simulink model "MissionManager"  (R2025b)
settings: Solver=FixedStepDiscrete  StartTime=0.0  StopTime=10  FixedStep=CMD_SAMPLE_TIME  RelTol=1e-3
undefined symbols (not defined in the file): CMD_SAMPLE_TIME
settings Model: DataDictionary=CommandDict.sldd  Creator=89447  LastModifiedBy=89447
settings OptimizationCC: DefaultParameterBehavior=Inlined  EnhancedBackFolding=on  PassReuseOutputArgsAs=Individual arguments  ZeroExternalMemoryAtStartup=off  ZeroInternalMemoryAtStartup=off  MaxStackSize=64  OptimizeBlockOrder=speed  DifferentSizesBufferReuse=on  OptimizationCustomize=off  EfficientTunableParamExpr=on
settings HardwareCC: ProdBitPerLong=64.0  ProdHWDeviceType=Intel->x86-64 (Linux 64)  TargetBitPerLong=64.0  TargetBitPerPointer=64.0  TargetBitPerSizeT=64.0  TargetBitPerPtrDiffT=64.0  TargetLargestAtomicFloat=Float  TargetIntDivRoundTo=Zero  TargetEndianess=LittleEndian  TargetWordSize=64.0  TargetHWDeviceType=Intel->x86-64 (Linux 64)  ProdEqTarget=off
settings SFSimCC: MATLABDynamicMemAlloc=off
settings RTWCC: SystemTargetFile=ert.tlc  HardwareBoard=Robot Operating System 2 (ROS 2)  TLCOptions="-aInlineSetEventsForThisBaseRateFcn=TLC_FALSE -aSuppressMultiTaskScheduler=TLC_FALSE  -aRateBasedStepFcn=0"  TemplateMakefile=ert_default_tmf  Toolchain=Colcon Tools  TargetLang=C++  Description=Embedded Coder
settings CodeAppCC: ForceParamTrailComments=on  IgnoreCustomStorageClasses=off  OperatorAnnotations=on  SimulinkDataObjDesc=on  SFDataObjDesc=on  InsertBlockDesc=on
settings ERTTargetCC: ExtModeTransport=2.0  ExtModeStaticAlloc=on  ExtModeMexFile=ext_xcp  ExtModeIntrfLevel=Level2 - Open  ERTCustomFileTemplate=example_file_process.tlc  TargetLangStandard=C++11 (ISO)  SupportContinuousTime=on

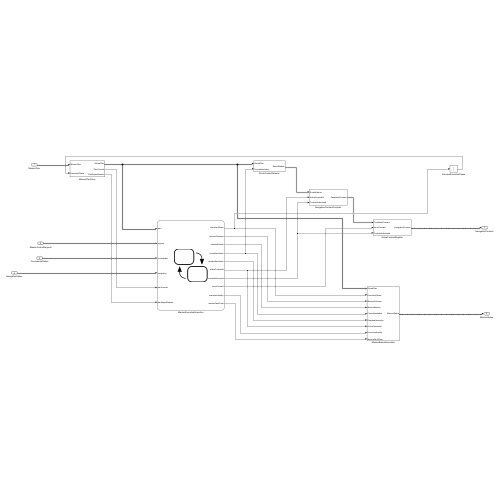
[thumbnail: Simulink's stored preview of the top-level diagram]
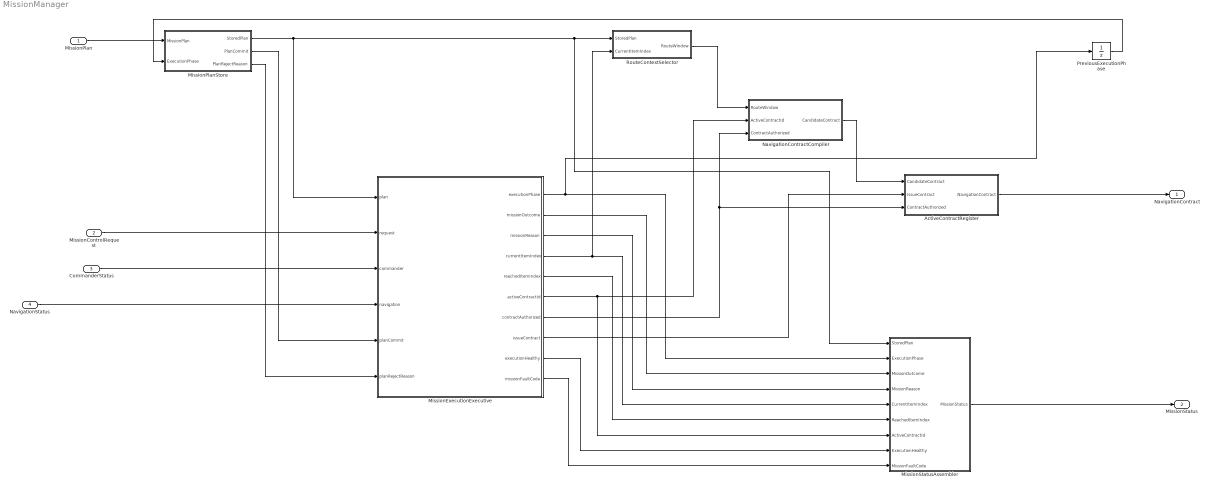
== system MissionManager ==
  MissionPlan : Inport  OutDataTypeStr=Bus: MissionPlanBus
  MissionControlRequest : Inport  Port=2  OutDataTypeStr=Bus: MissionControlRequestBus
  CommanderStatus : Inport  Port=3  OutDataTypeStr=Bus: CommanderStatusBus
  NavigationStatus : Inport  Port=4  OutDataTypeStr=Bus: NavigationStatusBus
  ActiveContractRegister : Subsystem
  MissionExecutionExecutive : Stateflow chart  TreatAsAtomicUnit=on
  MissionPlanStore : Subsystem
  MissionStatusAssembler : Subsystem
  NavigationContractCompiler : Subsystem
  PreviousExecutionPhase : UnitDelay  InitialCondition=uint8(0)  SampleTime=CMD_SAMPLE_TIME
  RouteContextSelector : Subsystem
  NavigationContract : Outport  OutDataTypeStr=Bus: NavigationContractBus
  MissionStatus : Outport  Port=2  OutDataTypeStr=Bus: MissionStatusBus
  wires:
  MissionPlan/1 -> MissionPlanStore/1(MissionPlan)
  MissionExecutionExecutive/1(executionPhase) -> MissionStatusAssembler/2(ExecutionPhase), PreviousExecutionPhase/1
  MissionPlanStore/1(StoredPlan) -> MissionStatusAssembler/1(StoredPlan), RouteContextSelector/1(StoredPlan), MissionExecutionExecutive/1(plan)
  MissionControlRequest/1 -> MissionExecutionExecutive/2(request)
  CommanderStatus/1 -> MissionExecutionExecutive/3(commander)
  NavigationStatus/1 -> MissionExecutionExecutive/4(navigation)
  MissionPlanStore/2(PlanCommit) -> MissionExecutionExecutive/5(planCommit)
  MissionPlanStore/3(PlanRejectReason) -> MissionExecutionExecutive/6(planRejectReason)
  MissionExecutionExecutive/4(currentItemIndex) -> MissionStatusAssembler/5(CurrentItemIndex), RouteContextSelector/2(CurrentItemIndex)
  RouteContextSelector/1(RouteWindow) -> NavigationContractCompiler/1(RouteWindow)
  MissionExecutionExecutive/6(activeContractId) -> NavigationContractCompiler/2(ActiveContractId), MissionStatusAssembler/7(ActiveContractId)
  MissionExecutionExecutive/7(contractAuthorized) -> NavigationContractCompiler/3(ContractAuthorized), ActiveContractRegister/3(ContractAuthorized)
  NavigationContractCompiler/1(CandidateContract) -> ActiveContractRegister/1(CandidateContract)
  MissionExecutionExecutive/8(issueContract) -> ActiveContractRegister/2(IssueContract)
  ActiveContractRegister/1(NavigationContract) -> NavigationContract/1
  MissionExecutionExecutive/2(missionOutcome) -> MissionStatusAssembler/3(MissionOutcome)
  MissionExecutionExecutive/3(missionReason) -> MissionStatusAssembler/4(MissionReason)
  MissionExecutionExecutive/5(reachedItemIndex) -> MissionStatusAssembler/6(ReachedItemIndex)
  MissionExecutionExecutive/9(executionHealthy) -> MissionStatusAssembler/8(ExecutionHealthy)
  MissionExecutionExecutive/10(missionFaultCode) -> MissionStatusAssembler/9(MissionFaultCode)
  MissionStatusAssembler/1(MissionStatus) -> MissionStatus/1
  PreviousExecutionPhase/1 -> MissionPlanStore/2(ExecutionPhase)

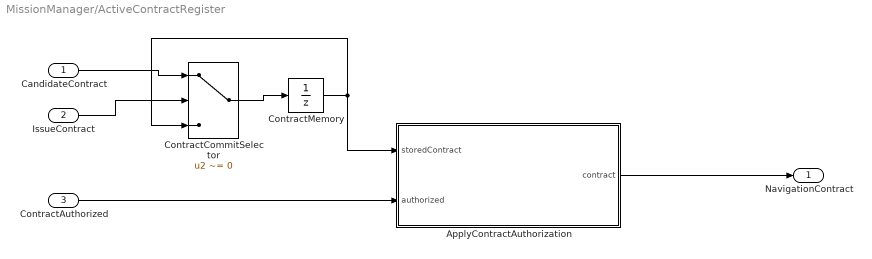
== system MissionManager/ActiveContractRegister ==
  CandidateContract : Inport  OutDataTypeStr=Bus: NavigationContractBus
  IssueContract : Inport  Port=2  OutDataTypeStr=boolean
  ContractAuthorized : Inport  Port=3  OutDataTypeStr=boolean
  ApplyContractAuthorization : MATLAB Function  TreatAsAtomicUnit=on
  ContractCommitSelector : Switch  Criteria=u2 ~= 0
  ContractMemory : UnitDelay  SampleTime=CMD_SAMPLE_TIME
  NavigationContract : Outport  OutDataTypeStr=Bus: NavigationContractBus
  wires:
  CandidateContract/1 -> ContractCommitSelector/1
  IssueContract/1 -> ContractCommitSelector/2
  ContractMemory/1 -> ApplyContractAuthorization/1(storedContract), ContractCommitSelector/3
  ContractCommitSelector/1 -> ContractMemory/1
  ContractAuthorized/1 -> ApplyContractAuthorization/2(authorized)
  ApplyContractAuthorization/1(contract) -> NavigationContract/1

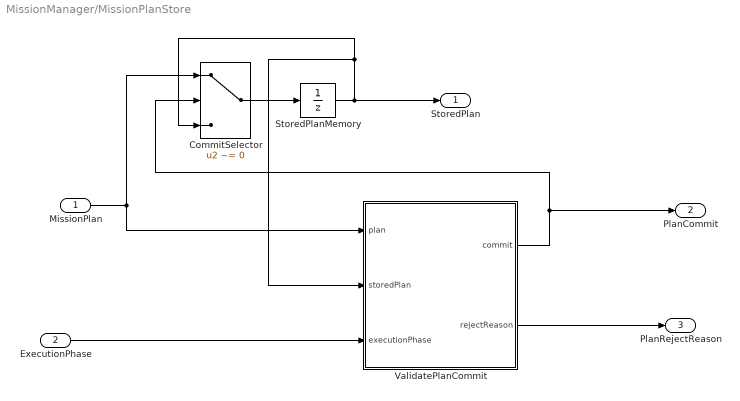
== system MissionManager/MissionPlanStore ==
  MissionPlan : Inport  OutDataTypeStr=Bus: MissionPlanBus
  ExecutionPhase : Inport  Port=2  OutDataTypeStr=uint8
  CommitSelector : Switch  Criteria=u2 ~= 0
  StoredPlanMemory : UnitDelay  SampleTime=CMD_SAMPLE_TIME
  ValidatePlanCommit : MATLAB Function  TreatAsAtomicUnit=on
  StoredPlan : Outport  OutDataTypeStr=Bus: MissionPlanBus
  PlanCommit : Outport  Port=2  OutDataTypeStr=boolean
  PlanRejectReason : Outport  Port=3  OutDataTypeStr=uint8
  wires:
  MissionPlan/1 -> ValidatePlanCommit/1(plan), CommitSelector/1
  StoredPlanMemory/1 -> CommitSelector/3, ValidatePlanCommit/2(storedPlan), StoredPlan/1
  ExecutionPhase/1 -> ValidatePlanCommit/3(executionPhase)
  ValidatePlanCommit/1(commit) -> PlanCommit/1, CommitSelector/2
  CommitSelector/1 -> StoredPlanMemory/1
  ValidatePlanCommit/2(rejectReason) -> PlanRejectReason/1

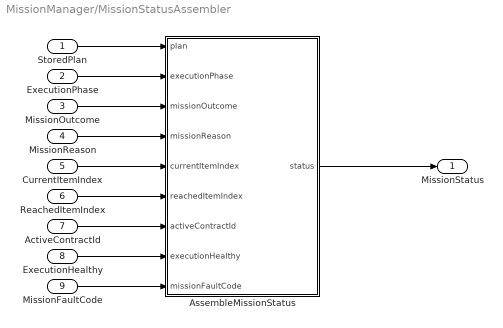
== system MissionManager/MissionStatusAssembler ==
  StoredPlan : Inport  OutDataTypeStr=Bus: MissionPlanBus
  ExecutionPhase : Inport  Port=2  OutDataTypeStr=uint8
  MissionOutcome : Inport  Port=3  OutDataTypeStr=uint8
  MissionReason : Inport  Port=4  OutDataTypeStr=uint8
  CurrentItemIndex : Inport  Port=5  OutDataTypeStr=uint8
  ReachedItemIndex : Inport  Port=6  OutDataTypeStr=int16
  ActiveContractId : Inport  Port=7  OutDataTypeStr=uint32
  ExecutionHealthy : Inport  Port=8  OutDataTypeStr=boolean
  MissionFaultCode : Inport  Port=9  OutDataTypeStr=uint16
  AssembleMissionStatus : MATLAB Function  TreatAsAtomicUnit=on
  MissionStatus : Outport  OutDataTypeStr=Bus: MissionStatusBus
  wires:
  StoredPlan/1 -> AssembleMissionStatus/1(plan)
  ExecutionPhase/1 -> AssembleMissionStatus/2(executionPhase)
  MissionOutcome/1 -> AssembleMissionStatus/3(missionOutcome)
  MissionReason/1 -> AssembleMissionStatus/4(missionReason)
  CurrentItemIndex/1 -> AssembleMissionStatus/5(currentItemIndex)
  ReachedItemIndex/1 -> AssembleMissionStatus/6(reachedItemIndex)
  ActiveContractId/1 -> AssembleMissionStatus/7(activeContractId)
  ExecutionHealthy/1 -> AssembleMissionStatus/8(executionHealthy)
  MissionFaultCode/1 -> AssembleMissionStatus/9(missionFaultCode)
  AssembleMissionStatus/1(status) -> MissionStatus/1

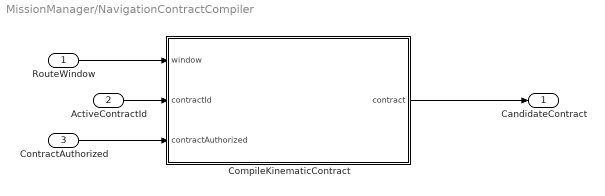
== system MissionManager/NavigationContractCompiler ==
  RouteWindow : Inport  OutDataTypeStr=Bus: RouteWindowBus
  ActiveContractId : Inport  Port=2  OutDataTypeStr=uint32
  ContractAuthorized : Inport  Port=3  OutDataTypeStr=boolean
  CompileKinematicContract : MATLAB Function  TreatAsAtomicUnit=on
  CandidateContract : Outport  OutDataTypeStr=Bus: NavigationContractBus
  wires:
  RouteWindow/1 -> CompileKinematicContract/1(window)
  ActiveContractId/1 -> CompileKinematicContract/2(contractId)
  ContractAuthorized/1 -> CompileKinematicContract/3(contractAuthorized)
  CompileKinematicContract/1(contract) -> CandidateContract/1

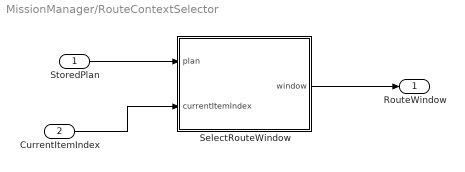
== system MissionManager/RouteContextSelector ==
  StoredPlan : Inport  OutDataTypeStr=Bus: MissionPlanBus
  CurrentItemIndex : Inport  Port=2  OutDataTypeStr=uint8
  SelectRouteWindow : MATLAB Function  TreatAsAtomicUnit=on
  RouteWindow : Outport  OutDataTypeStr=Bus: RouteWindowBus
  wires:
  StoredPlan/1 -> SelectRouteWindow/1(plan)
  CurrentItemIndex/1 -> SelectRouteWindow/2(currentItemIndex)
  SelectRouteWindow/1(window) -> RouteWindow/1

== matlab function MissionManager/MissionStatusAssembler/AssembleMissionStatus ==
  data: plan input; status output Bus: MissionStatusBus; executionPhase input; missionOutcome input; missionReason input; currentItemIndex input; reachedItemIndex input; activeContractId input; executionHealthy input; missionFaultCode input
function status = AssembleMissionStatus(plan, executionPhase, missionOutcome, missionReason, currentItemIndex, reachedItemIndex, activeContractId, executionHealthy, missionFaultCode)
% Assemble observation-only mission status from authoritative facts.
status.PlanId = plan.PlanId;
status.PlanValid = plan.Valid;
status.ExecutionPhase = executionPhase;
status.MissionOutcome = missionOutcome;
status.MissionReason = missionReason;
status.CurrentItemIndex = currentItemIndex;
status.ItemCount = plan.ItemCount;
status.ReachedItemIndex = reachedItemIndex;
status.ActiveContractId = activeContractId;
status.ExecutionHealthy = executionHealthy;
status.MissionFaultCode = missionFaultCode;
status.LandingCompleted = false;
if plan.Valid && executionPhase == uint8(3) && missionOutcome == uint8(1) && ...
        plan.ItemCount > uint8(0) && currentItemIndex < plan.ItemCount
    itemIndex = double(currentItemIndex) + 1.0;
    status.LandingCompleted = plan.ItemType(itemIndex) == uint8(3);
end
status.Valid = true;
end

== matlab function MissionManager/RouteContextSelector/SelectRouteWindow ==
  data: plan input; window output Bus: RouteWindowBus; currentItemIndex input
function window = SelectRouteWindow(plan, currentItemIndex)
% Select Previous/Current/Next only from the immutable stored plan.
window.PlanId = uint32(0);
window.ItemIndex = currentItemIndex;
window.PreviousValid = false;
window.PreviousPositionNED = zeros(3,1,'single');
window.CurrentTaskType = uint8(0);
window.CurrentPositionNED = zeros(3,1,'single');
window.CurrentYaw = single(0);
window.AcceptanceRadius = single(0);
window.TerminalBehavior = uint8(0);
window.AdvancePolicy = uint8(0);
window.DwellTime = single(0);
window.CruiseSpeed = single(0);
window.MaxAcceleration = single(0);
window.MaxJerk = single(0);
window.NextValid = false;
window.NextPositionNED = zeros(3,1,'single');
window.IsFirstItem = false;
window.IsLastItem = false;
window.Valid = false;
if ~plan.Valid || plan.ItemCount < uint8(1)
    return;
end
count = double(plan.ItemCount);
idx = double(currentItemIndex) + 1.0;
if idx < 1.0 || idx > count || idx > 10.0
    return;
end
window.PlanId = plan.PlanId;
window.CurrentTaskType = plan.ItemType(idx);
window.CurrentPositionNED = reshape(plan.TargetPositionNED(idx,:),[3 1]);
window.CurrentYaw = plan.TargetYaw(idx);
window.AcceptanceRadius = plan.AcceptanceRadius(idx);
window.TerminalBehavior = plan.TerminalBehavior(idx);
window.AdvancePolicy = plan.AdvancePolicy(idx);
window.DwellTime = plan.DwellTime(idx);
window.CruiseSpeed = plan.CruiseSpeed(idx);
window.MaxAcceleration = plan.MaxAcceleration(idx);
window.MaxJerk = plan.MaxJerk(idx);
window.IsFirstItem = idx == 1.0;
window.IsLastItem = idx == count;
if idx > 1.0
    window.PreviousValid = true;
    window.PreviousPositionNED = reshape(plan.TargetPositionNED(idx-1.0,:),[3 1]);
end
if idx < count
    window.NextValid = true;
    window.NextPositionNED = reshape(plan.TargetPositionNED(idx+1.0,:),[3 1]);
end
window.Valid = true;
end

== matlab function MissionManager/MissionPlanStore/ValidatePlanCommit ==
  data: plan input; commit output; storedPlan input; executionPhase input; rejectReason output
function [commit, rejectReason] = ValidatePlanCommit(plan, storedPlan, executionPhase)
% Validate a complete fixed-capacity plan before one-time storage.
commit = false;
rejectReason = uint8(0);
if ~plan.Valid
    return;
end
if plan.PlanId == uint32(0)
    rejectReason = uint8(1);
    return;
end
if executionPhase == uint8(1) || executionPhase == uint8(2)
    rejectReason = uint8(2);
    return;
end
if storedPlan.Valid && plan.PlanId == storedPlan.PlanId
    return;
end
count = double(plan.ItemCount);
if count < 1 || count > 10
    rejectReason = uint8(3);
    return;
end
for k = 1:count
    if plan.ItemType(k) < uint8(1) || plan.ItemType(k) > uint8(3)
        rejectReason = uint8(4);
        return;
    end
    if any(~isfinite(plan.TargetPositionNED(k,:))) || ...
            ~isfinite(plan.TargetYaw(k)) || ...
            ~isfinite(plan.AcceptanceRadius(k)) || ...
            ~isfinite(plan.DwellTime(k)) || ...
            ~isfinite(plan.CruiseSpeed(k)) || ...
            ~isfinite(plan.MaxAcceleration(k)) || ...
            ~isfinite(plan.MaxJerk(k))
        rejectReason = uint8(5);
        return;
    end
    if plan.AcceptanceRadius(k) <= single(0) || ...
            plan.CruiseSpeed(k) < single(0) || ...
            plan.MaxAcceleration(k) < single(0) || ...
            plan.MaxJerk(k) < single(0)
        rejectReason = uint8(6);
        return;
    end
    if plan.TerminalBehavior(k) > uint8(2) || plan.AdvancePolicy(k) > uint8(1)
        rejectReason = uint8(7);
        return;
    end
    if plan.TerminalBehavior(k) == uint8(2)
        if plan.DwellTime(k) <= single(0)
            rejectReason = uint8(8);
            return;
        end
    elseif plan.DwellTime(k) ~= single(0)
        rejectReason = uint8(9);
        return;
    end
end
if plan.TerminalBehavior(count) == uint8(1)
    rejectReason = uint8(10);
    return;
end
commit = true;
end

== stateflow chart MissionManager/MissionExecutionExecutive ==
  state IDLE
    entry:
    executionPhase = uint8(0);
    contractAuthorized = false;
    issueContract = false;
    during:
    issueContract = false;
    if planCommit
    missionOutcome = uint8(0);
    missionReason = uint8(0);
    currentItemIndex = uint8(0);
    reachedItemIndex = int16(-1);
    executionHealthy = true;
    missionFaultCode = uint16(0);
    end
  state ACTIVE
    entry:
    executionPhase = uint8(1);
    contractAuthorized = true;
    issueContract = true;
    during:
    issueContract = false;
    if commander.Valid && commander.MissionDirective == uint8(0) && ...
    navigation.Valid && ...
    navigation.ContractId == activeContractId && ...
    navigation.TerminalConditionSatisfied && ...
    currentItemIndex + uint8(1) < plan.ItemCount && ...
    plan.AdvancePolicy(double(currentItemIndex)+1) == uint8(1)
    reachedItemIndex = int16(currentItemIndex);
    currentItemIndex = currentItemIndex + uint8(1);
    activeContractId = activeContractId + uint32(1);
    issueContract = true;
    end
  state SUSPENDED
    entry:
    executionPhase = uint8(2);
    contractAuthorized = false;
    issueContract = false;
    during:
    issueContract = false;
  state ENDED
    entry:
    executionPhase = uint8(3);
    issueContract = false;
    contractAuthorized = missionOutcome == uint8(1);
    during:
    issueContract = false;
  (default) -> IDLE : {missionOutcome=uint8(0); missionReason=uint8(0); currentItemIndex=uint8(0); reachedItemIndex=int16(-1); activeContractId=uint32(0); executionHealthy=true; missionFaultCode=uint16(0); lastRequestId=intmax('uint32');}
  IDLE -> ACTIVE : [plan.Valid && request.Valid && request.RequestId ~= lastRequestId && ...
      |  request.Action == uint8(1) && (request.PlanId == uint32(0) || request.PlanId == plan.PlanId) && ...
      |  commander.Valid && commander.Armed && commander.MissionExecutionAllowed && ...
      |  commander.MissionDirective == uint8(0) && ~commander.FailsafeActive]
      | {lastRequestId=request.RequestId; missionOutcome=uint8(0); missionReason=uint8(0); currentItemIndex=uint8(0); reachedItemIndex=int16(-1); activeContractId=activeContractId+uint32(1); executionHealthy=true; missionFaultCode=uint16(0);}
  ENDED -> IDLE : [planCommit]
  ACTIVE -> SUSPENDED [order 3] : [request.Valid && request.RequestId ~= lastRequestId && request.Action == uint8(2)]
      | {lastRequestId=request.RequestId; missionReason=uint8(3);}
  ACTIVE -> SUSPENDED [order 4] : [commander.MissionDirective ~= uint8(2) && ...
      |  (~commander.Valid || ~commander.Armed || ...
      |   ~commander.MissionExecutionAllowed || commander.FailsafeActive || ...
      |   commander.MissionDirective == uint8(1))]
      | {missionReason=uint8(5);}
  ACTIVE -> SUSPENDED [order 5] : [~plan.Valid || currentItemIndex >= plan.ItemCount]
      | {missionReason=uint8(6); executionHealthy=false; missionFaultCode=uint16(1);}
  ACTIVE -> SUSPENDED [order 7] : [commander.Valid && commander.MissionDirective == uint8(0) && ...
      |  navigation.Valid && navigation.ContractId == activeContractId && ...
      |  navigation.TerminalConditionSatisfied && currentItemIndex + uint8(1) < plan.ItemCount && ...
      |  plan.AdvancePolicy(double(currentItemIndex)+1) == uint8(0)]
      | {reachedItemIndex=int16(currentItemIndex); currentItemIndex=currentItemIndex+uint8(1); missionReason=uint8(4);}
  SUSPENDED -> ACTIVE [order 2] : [request.Valid && request.RequestId ~= lastRequestId && request.Action == uint8(3) && ...
      |  plan.Valid && commander.Valid && commander.Armed && ...
      |  commander.MissionExecutionAllowed && commander.MissionDirective == uint8(0) && ...
      |  ~commander.FailsafeActive && executionHealthy]
      | {lastRequestId=request.RequestId; missionReason=uint8(0); activeContractId=activeContractId+uint32(1);}
  ACTIVE -> ENDED [order 6] : [commander.Valid && commander.MissionDirective == uint8(0) && ...
      |  navigation.Valid && navigation.ContractId == activeContractId && ...
      |  navigation.TerminalConditionSatisfied && currentItemIndex + uint8(1) >= plan.ItemCount]
      | {reachedItemIndex=int16(currentItemIndex); missionOutcome=uint8(1); missionReason=uint8(1);}
  ACTIVE -> ENDED [order 1] : [commander.Valid && commander.MissionDirective == uint8(2)]
      | {missionOutcome=uint8(3); missionReason=uint8(7); contractAuthorized=false;}
  ACTIVE -> ENDED [order 2] : [request.Valid && request.RequestId ~= lastRequestId && request.Action == uint8(4)]
      | {lastRequestId=request.RequestId; missionOutcome=uint8(2); missionReason=uint8(2); contractAuthorized=false;}
  SUSPENDED -> ENDED [order 3] : [request.Valid && request.RequestId ~= lastRequestId && request.Action == uint8(4)]
      | {lastRequestId=request.RequestId; missionOutcome=uint8(2); missionReason=uint8(2);}
  SUSPENDED -> ENDED [order 1] : [commander.Valid && commander.MissionDirective == uint8(2)]
      | {missionOutcome=uint8(3); missionReason=uint8(7); contractAuthorized=false;}
  data: plan input Bus: MissionPlanBus; request input Bus: MissionControlRequestBus; commander input Bus: CommanderStatusBus; navigation input Bus: NavigationStatusBus; planCommit input boolean; planRejectReason input uint8; executionPhase output uint8; missionOutcome output uint8; missionReason output uint8; currentItemIndex output uint8; reachedItemIndex output int16; activeContractId output uint32; contractAuthorized output boolean; issueContract output boolean; executionHealthy output boolean; missionFaultCode output uint16; lastRequestId local uint32

== matlab function MissionManager/NavigationContractCompiler/CompileKinematicContract ==
  data: window input; contract output Bus: NavigationContractBus; contractId input; contractAuthorized input
function contract = CompileKinematicContract(window, contractId, contractAuthorized)
% Compile one task-neutral contract from the active stored-plan window.
contract.ContractId = contractId;
contract.PlanId = window.PlanId;
contract.ItemIndex = window.ItemIndex;
contract.PathType = uint8(1);
contract.SegmentStartValid = window.PreviousValid;
contract.SegmentStartPositionNED = window.PreviousPositionNED;
contract.SegmentEndPositionNED = window.CurrentPositionNED;
contract.TerminalVelocityNED = zeros(3,1,'single');
contract.ExitDirectionNED = zeros(3,1,'single');
contract.CruiseSpeed = window.CruiseSpeed;
contract.MaxAcceleration = window.MaxAcceleration;
contract.MaxJerk = window.MaxJerk;
contract.TargetYaw = window.CurrentYaw;
contract.AcceptanceRadius = window.AcceptanceRadius;
contract.RequiredStableTime = single(0);
contract.Valid = false;
if ~window.Valid || ~contractAuthorized
    return;
end
flyThrough = window.TerminalBehavior == uint8(1) && ...
    window.NextValid && ~window.IsLastItem;
if flyThrough
    outgoing = window.NextPositionNED - window.CurrentPositionNED;
    outgoingNorm = sqrt(sum(outgoing .* outgoing));
    if outgoingNorm > single(1.0e-6)
        direction = outgoing / outgoingNorm;
        contract.ExitDirectionNED = direction;
        contract.TerminalVelocityNED = window.CruiseSpeed * direction;
    end
elseif window.TerminalBehavior == uint8(2)
    contract.RequiredStableTime = window.DwellTime;
end
contract.Valid = true;
end

== matlab function MissionManager/ActiveContractRegister/ApplyContractAuthorization ==
  data: storedContract input; contract output Bus: NavigationContractBus; authorized input
function contract = ApplyContractAuthorization(storedContract, authorized)
% Preserve immutable contract content while independently gating execution.
contract = storedContract;
contract.Valid = storedContract.Valid && authorized;
end
